simulink model "controlTuning"  (R2022b)
settings: Solver=VariableStepAuto  StartTime=0.0  StopTime=1000  RelTol=1e-12
undefined symbols (not defined in the file or in its folder): sat, settings
libraries: matrix_library x1
settings Model: Creator=brent  LastModifiedBy=brent

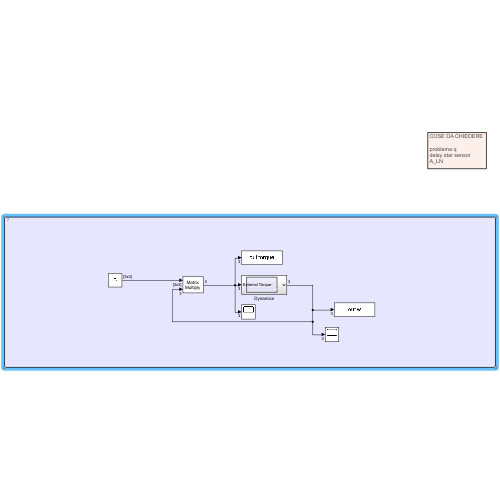
[thumbnail: Simulink's stored preview of the top-level diagram]
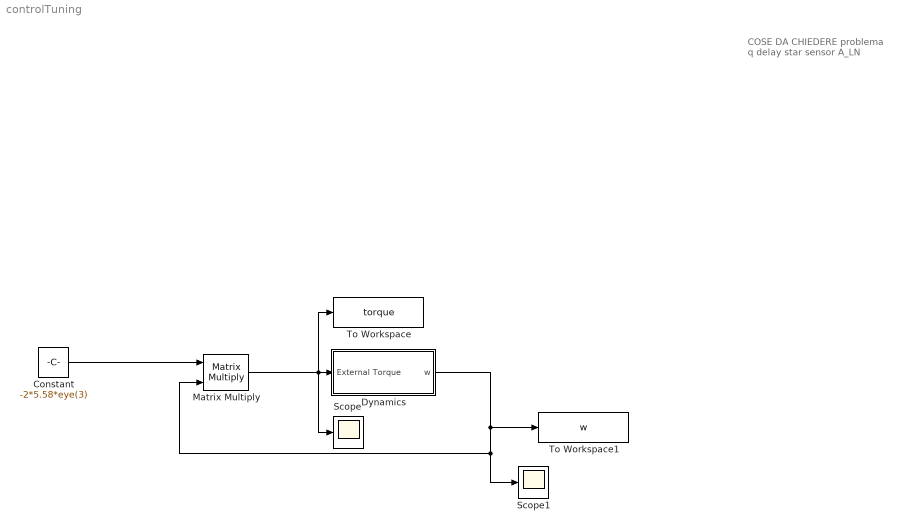
== system controlTuning ==
  note: COSE DA CHIEDERE
      |
      | problema q
      | delay star sensor
      | A_LN
  Constant : Constant  Value=-2*5.58*eye(3)
  Dynamics : Subsystem
  Matrix Multiply : Product  Multiplication=Matrix(*)
  Scope : Scope
  Scope1 : Scope
  To Workspace : ToWorkspace  VariableName=torque  SampleTime=-1
  To Workspace1 : ToWorkspace  VariableName=w  SampleTime=-1
  wires:
  Dynamics/1(w) -> To Workspace1/1, Scope1/1, Matrix Multiply/2
  Constant/1 -> Matrix Multiply/1
  Matrix Multiply/1 -> Scope/1, To Workspace/1, Dynamics/1(External Torque)

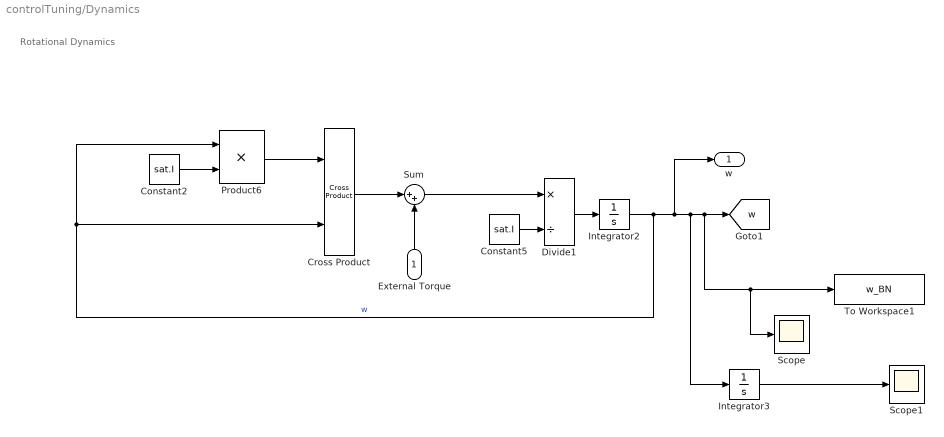
== system controlTuning/Dynamics ==
  note: Rotational Dynamics
  External Torque : Inport
  Constant2 : Constant  Value=sat.I
  Constant5 : Constant  Value=sat.I
  Cross Product : matrix_library/Cross Product
  Divide1 : Product  Inputs=*/
  Integrator2 : Integrator  InitialCondition=settings.w0
  Integrator3 : Integrator  InitialCondition=[0 0 0]
  Product6 : Product
  Scope : Scope
  Scope1 : Scope
  Sum : Sum  Inputs=|++
  To Workspace1 : ToWorkspace  VariableName=w_BN  SampleTime=-1
  w : Outport
  tag scope: w=global
  wires:
  Divide1/1 -> Integrator2/1
  Sum/1 -> Divide1/1
  Product6/1 -> Cross Product/1
  Integrator2/1 -> Cross Product/2, Product6/1, Integrator3/1, To Workspace1/1, Scope/1, [w], w/1  "w"
  Constant2/1 -> Product6/2
  Cross Product/1 -> Sum/1
  Constant5/1 -> Divide1/2
  External Torque/1 -> Sum/2
  Integrator3/1 -> Scope1/1
